simulink model "Bai03"  (R2023b)
settings: Solver=VariableStepAuto  StartTime=0.0  StopTime=0.5  RelTol=1e-3
settings Model: Creator=Trung  LastModifiedBy=Trung

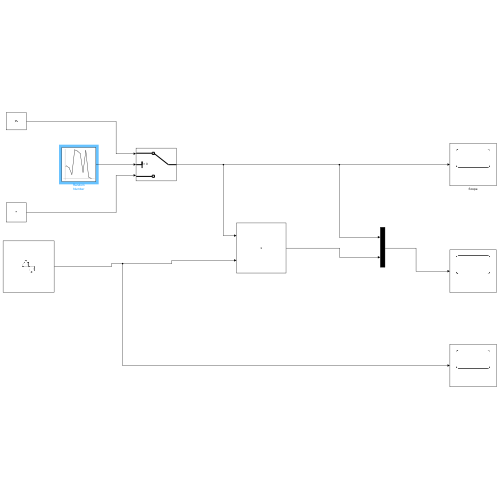
[thumbnail: Simulink's stored preview of the top-level diagram]
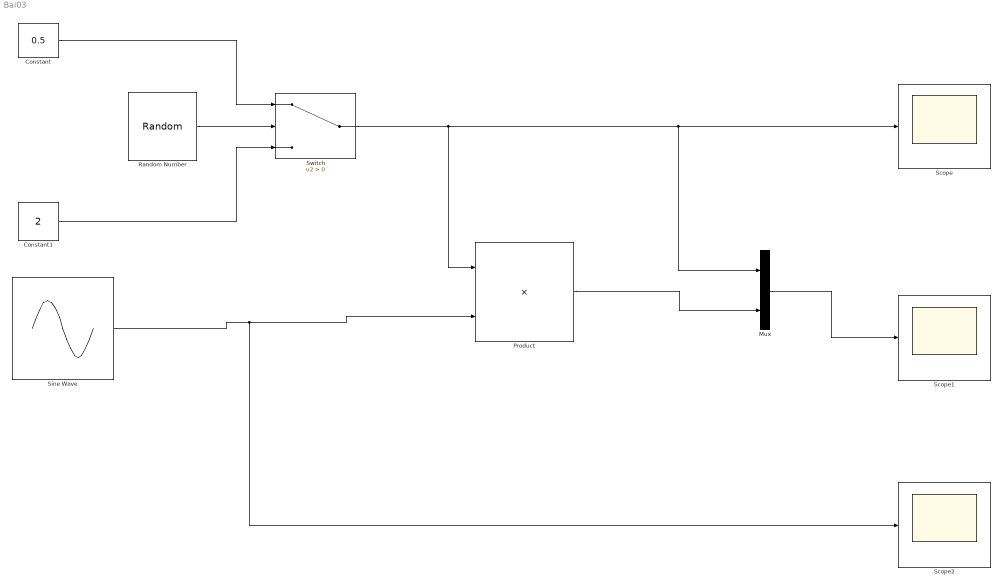
== system Bai03 ==
  Constant : Constant  Value=0.5
  Constant1 : Constant  Value=2
  Mux : Mux  Inputs=2
  Product : Product
  Random Number : RandomNumber  Seed=10  SampleTime=0.1  VectorParams1D=off
  Scope : Scope
  Scope1 : Scope
  Scope2 : Scope
  Sine Wave : Sin  Frequency=40*pi  SampleTime=0.00001
  Switch : Switch  Criteria=u2 > Threshold  SaturateOnIntegerOverflow=off  InputSameDT=off
  wires:
  Constant/1 -> Switch/1
  Random Number/1 -> Switch/2
  Constant1/1 -> Switch/3
  Switch/1 -> Product/1, Mux/1, Scope/1
  Sine Wave/1 -> Scope2/1, Product/2
  Product/1 -> Mux/2
  Mux/1 -> Scope1/1
